simulink model "identification"  (R2024b)
settings: Solver=FixedStepAuto  StartTime=0.0  StopTime=40  RelTol=1e-3  EnableMultiTasking=on
libraries: Blokk_Konyvtar x2, simulink x1
settings Model: STM32="{\"HardwareInterrupt\":[{\"ID\":\"untitled:2:120\"},{\"ID\":\"identification:13:120\"}],\"DigitalPortRead\":[{\"ID\":\"untitled:2:28\"},{\"ID\":\"untitled:2:29\"},{\"ID\":\"untitled:2:56\"},{\"ID\":\"untitled:2:57\"},{\"ID\":\"untitled:2:80\"},{\"ID\":\"untitled:2:81\"},{\"ID\":\"untitled:2:108\"},{\"ID\":\"untitled:2:109\"},{\"ID\":\"identification:13:28\"},{\"ID\":\"identification:13:29\"},{\"ID\":\"identification:13:56\"},{\"ID\":\"identification:13:57\"},{\"ID\":\"identification:13:80\"},{\"ID\":\"identification:13:81\"},{\"ID\":\"identification:13:108\"},{\"ID\":\"identification:13:109\"}],\"TimerCapture\":[{\"ID\":\"untitled:2:39\"},{\"ID\":\"untitled:2:91\"},{\"ID\":\"identification:13:39\"},{\"ID\":\"identification:13:91\"}],\"PWMOutput\":[{\"ID\":\"untitled:1:211\"},{\"ID\":\"untitled:1:212\"},{\"ID\":\"untitled:1:217\"},{\"ID\":\"untitled:1:218\"},{\"ID\":\"identification:1:217\"},{\"ID\":\"identification:1:218\"}],\"DigitalPortWrite\":[{\"ID\":\"untitled:1:219\"},{\"ID\":\"identification:1:219\"}]}"  Creator=Asus  LastModifiedBy=Asus
settings OptimizationCC: DefaultParameterBehavior=Inlined  EnhancedBackFolding=on  PassReuseOutputArgsAs=Individual arguments  ZeroExternalMemoryAtStartup=off  ZeroInternalMemoryAtStartup=off  MaxStackSize=512  OptimizeBlockOrder=speed  DifferentSizesBufferReuse=on  OptimizationCustomize=off  EfficientTunableParamExpr=on
settings DebuggingCC: TasksWithSamePriorityMsg=none  ParameterTunabilityLossMsg=error
settings HardwareCC: ProdBitPerPointer=32  ProdBitPerSizeT=32  ProdBitPerPtrDiffT=32  ProdLargestAtomicInteger=Long  ProdLargestAtomicFloat=Double  ProdWordSize=32  ProdLongLongMode=on  ProdHWDeviceType=ARM Compatible->ARM Cortex-M
settings SFSimCC: MATLABDynamicMemAlloc=off
settings RTWCC: Description=Embedded Coder  SystemTargetFile=ert.tlc  HardwareBoard=STM32F4xx Based  TemplateMakefile=ert_default_tmf  Toolchain=GNU Tools for ARM Embedded Processors
settings CodeAppCC: ForceParamTrailComments=on  IgnoreCustomStorageClasses=off  OperatorAnnotations=on  SimulinkDataObjDesc=on  SFDataObjDesc=on  InsertBlockDesc=on
settings ERTTargetCC: TargetLangStandard=C99 (ISO)  CodeReplacementLibrary=ARM Cortex-M  ExtModeTransport=3  ExtModeStaticAlloc=on  ExtModeStaticAllocSize=2048  ExtModeMexFile=ext_xcp  ExtModeIntrfLevel=Level2 - Open

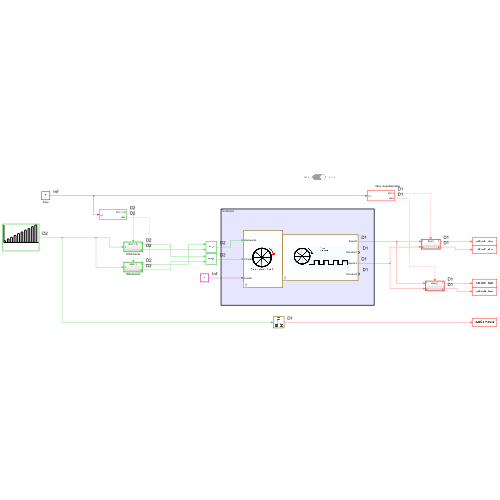
[thumbnail: Simulink's stored preview of the top-level diagram]
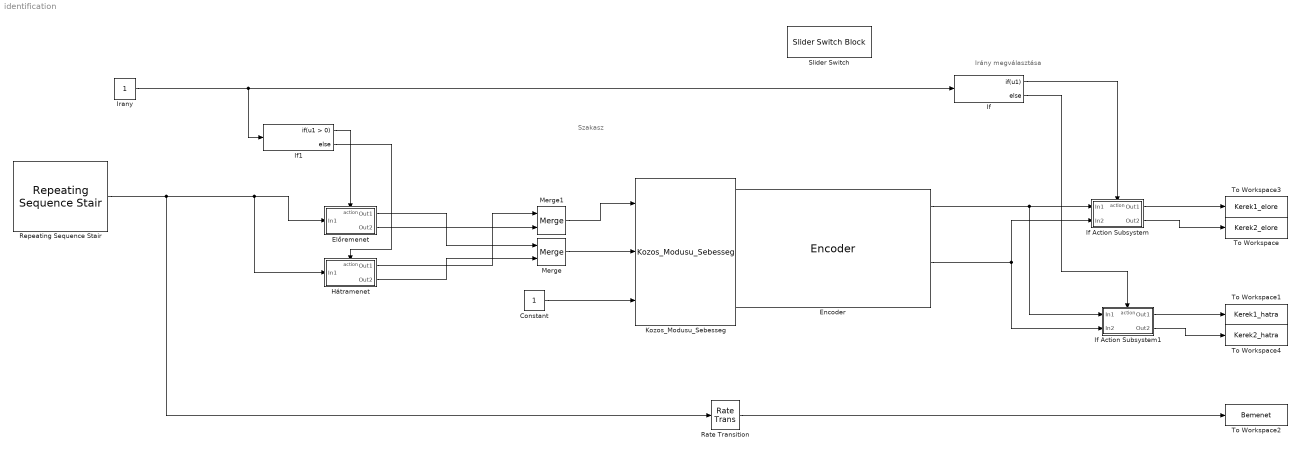
== system identification ==
  note: Irány megválasztása
  note: Szakasz
  Constant : Constant
  Előremenet : Subsystem  TreatAsAtomicUnit=on
  Encoder : Blokk_Konyvtar/Encoder  TimClkFrq=25e6  CPR=1024  fwdvalue1=0  fwdvalue2=1  bckvalue1=1  bckvalue2=0  PrScaler=1
      settings: SourceProductName=Blokk_Konyvtar
  Hátramenet : Subsystem  TreatAsAtomicUnit=on
  If : If  IfExpression=u1
  If Action Subsystem : Subsystem  TreatAsAtomicUnit=on
  If Action Subsystem1 : Subsystem  TreatAsAtomicUnit=on
  If1 : If
  Irany : Constant
  Kozos_Modusu_Sebesseg : Blokk_Konyvtar/Kozos_Modusu_Sebesseg
      settings: SourceProductName=Blokk_Konyvtar
  Merge : Merge
  Merge1 : Merge
  Rate Transition : RateTransition  Integrity=off  OutPortSampleTime=0.02
  Repeating Sequence Stair : simulink/Sources/Repeating Sequence Stair  OutValues=[10 0 20 0 30 0 40 0 50 0 60 0 70 0 80 0 90 0 99 0].'  tsamp=2  OutMin=[]  OutMax=[]  OutDataTypeStr=double  OutputDataTypeScalingMode=double  OutDataType=fixdt(0,8)  ConRadixGroup=Best Precision: Vector-wise  OutScaling=2^-12
  Slider Switch : SliderSwitchBlock  LabelPosition=Hide
      settings: Values={{'Hatra', 'Elore'}, [0 1]}
  To Workspace : ToWorkspace  VariableName=Kerek2_elore  SaveFormat=Timeseries  SampleTime=-1
  To Workspace1 : ToWorkspace  VariableName=Kerek1_hatra  SaveFormat=Timeseries  SampleTime=-1
  To Workspace2 : ToWorkspace  VariableName=Bemenet  SaveFormat=Timeseries  SampleTime=-1
  To Workspace3 : ToWorkspace  VariableName=Kerek1_elore  SaveFormat=Timeseries  SampleTime=-1
  To Workspace4 : ToWorkspace  VariableName=Kerek2_hatra  SaveFormat=Timeseries  SampleTime=-1
  wires:
  Encoder/3 -> If Action Subsystem1/2(In2), If Action Subsystem/2(In2)
  Encoder/1 -> If Action Subsystem1/1(In1), If Action Subsystem/1(In1)
  Constant/1 -> Kozos_Modusu_Sebesseg/3
  Repeating Sequence Stair/1 -> Rate Transition/1, Hátramenet/1(In1), Előremenet/1(In1)
  Előremenet/1(Out1) -> Merge/1
  Rate Transition/1 -> To Workspace2/1
  Irany/1 -> If/1, If1/1
  If Action Subsystem/1(Out1) -> To Workspace3/1
  If Action Subsystem/2(Out2) -> To Workspace/1
  If Action Subsystem1/1(Out1) -> To Workspace1/1
  If Action Subsystem1/2(Out2) -> To Workspace4/1
  If/1 -> If Action Subsystem/Action
  If/2 -> If Action Subsystem1/Action
  Hátramenet/1(Out1) -> Merge1/1
  Hátramenet/2(Out2) -> Merge/2
  Előremenet/2(Out2) -> Merge1/2
  Merge1/1 -> Kozos_Modusu_Sebesseg/1
  Merge/1 -> Kozos_Modusu_Sebesseg/2
  If1/1 -> Előremenet/Action
  If1/2 -> Hátramenet/Action

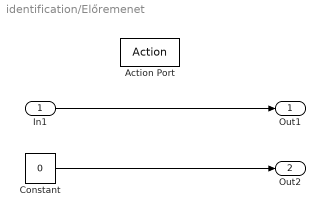
== system identification/Előremenet ==
  In1 : Inport
  Action Port : ActionPort  ActionPortLabel=if(u1 > 0)
  Constant : Constant  Value=0
  Out1 : Outport
  Out2 : Outport  Port=2
  wires:
  In1/1 -> Out1/1
  Constant/1 -> Out2/1

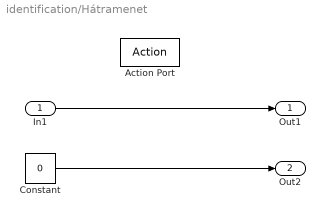
== system identification/Hátramenet ==
  In1 : Inport
  Action Port : ActionPort  ActionPortLabel=else
  Constant : Constant  Value=0
  Out1 : Outport
  Out2 : Outport  Port=2
  wires:
  In1/1 -> Out1/1
  Constant/1 -> Out2/1

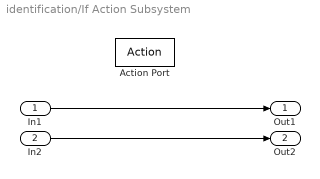
== system identification/If Action Subsystem ==
  In1 : Inport
  In2 : Inport  Port=2
  Action Port : ActionPort  ActionPortLabel=if(u1)
  Out1 : Outport
  Out2 : Outport  Port=2
  wires:
  In1/1 -> Out1/1
  In2/1 -> Out2/1

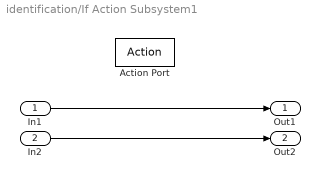
== system identification/If Action Subsystem1 ==
  In1 : Inport
  In2 : Inport  Port=2
  Action Port : ActionPort  ActionPortLabel=else
  Out1 : Outport
  Out2 : Outport  Port=2
  wires:
  In1/1 -> Out1/1
  In2/1 -> Out2/1
